simulink model "FB_Controller"  (R2018b)
settings: Solver=FixedStepDiscrete  StartTime=0.0  StopTime=50  FixedStep=1  MaxStep=1  RelTol=1e-3
values from neighbouring files (symbols this model uses):
  read_input_code = uint8(2)    [setup.m]
  timeout = int32(50)    [setup.m]
  write_output_code = uint8(4)    [setup.m]
undefined symbols (not defined in the file or in its folder): sldvsubsys
libraries: sldvlib x11, simulink x4, hdlsllib x3, simulink_extras x1
settings Model: PauseTimes=16.5  Creator=gauthamsm  LastModifiedBy=gauthamsm
settings DebuggingCC: IntegerOverflowMsg=error  IntegerSaturationMsg=error
settings ConfigComp: DVMode=PropertyProving  DVTestSuiteOptimization=CombinedObjectives (Nonlinear Extended)  DVDetectOutOfBounds=on

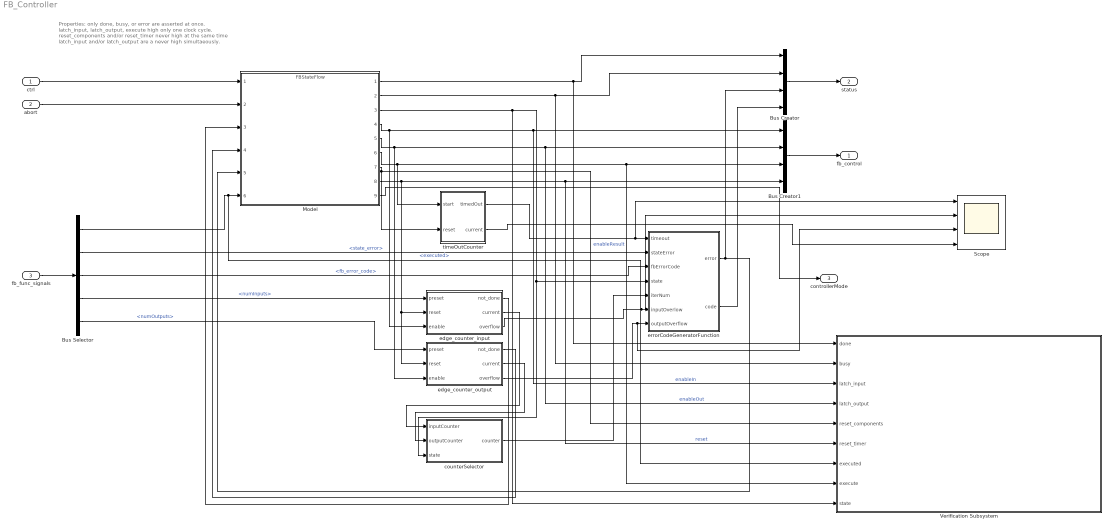
== system FB_Controller ==
  note: Properties:
      | only done, busy, or error are asserted at once.
      | latch_input, latch_output, execute high only one clock cycle.
      | reset_components and/or reset_timer never high at the same time latch_input and/or latch_output are a never high simultaeously.
  ctrl : Inport  RequirementInfo={} %GIDa_eee56b84_8a81_4d0c_8bf5_519b6d3ee13a  OutDataTypeStr=boolean
  abort : Inport  RequirementInfo={} %GIDa_f7a011da_777c_48fa_ab6a_d93ba2b9ac0e  Port=2  OutDataTypeStr=boolean
  fb_func_signals : Inport  RequirementInfo={} %GIDa_558a3938_4bec_4c5e_9357_eecde6866582  Port=3  OutDataTypeStr=Bus: fb_functions_out
  Bus Creator : BusCreator  RequirementInfo={} %GIDa_5b43234e_00ef_49d3_92d1_0649bce15cf8  Inputs=4  OutDataTypeStr=Bus: fb_status
  Bus Creator1 : BusCreator  RequirementInfo={} %GIDa_2879ab44_2c47_481b_b9a6_000ecd94b36b  Inputs=4  OutDataTypeStr=Bus: fb_control
  Bus Selector : BusSelector  RequirementInfo={} %GIDa_3f3a83a6_ae23_41f2_94a0_96f7ad6d1f78  OutputSignals=executed,state_error,fb_error_code,numInputs,numOutputs
  Model : ModelReference  RequirementInfo={} %GIDa_1daab9a8_dd2d_4e6d_9772_3109c5418e4f  ModelNameDialog=FBStateFlow.slx  SimulationMode=Normal  ModelReferenceVersion=1.25
  Scope : Scope  NumInputPorts=4
  Verification Subsystem : Subsystem  Tag=VerificationSubsystem  DisableCoverage=on  LoadFcn=sldvsubsys('check')  TreatAsAtomicUnit=on  SimViewingDevice=on  mask(VerificationSubsystem){}
      mask init:
      | sldvsubsys('maskInit');
      settings: CopyFcn=sldvsubsys('copy');  OpenFcn=open_system(gcb,'force');
      settings: PreSaveFcn=|
      | set_param(gcb,'SimViewingDevice','on');
      | sldvsubsys('check');
      mask Help: helpview(fullfile(docroot,'toolbox','sldv','sldv.map'),'verificationsubsystem')
      mask Display: image(imread('sldvicon_versubsys.png','BackGroundColor',[1 1 1]),'center');
  counterSelector : Subsystem  RequirementInfo={} %GIDa_611b34ef_a88f_49be_a0b4_a9f7defa758a  AncestorBlock=library/edge_counter
  edge_counter_input : Subsystem  AncestorBlock=library/edge_counter
  edge_counter_output : Subsystem  RequirementInfo={} %GIDa_3d032f53_0e8b_43fd_9dc3_9847963cb929  AncestorBlock=library/edge_counter
  errorCodeGeneratorFunction : Subsystem  RequirementInfo={} %GIDa_45c906d4_d4b7_4067_a1e4_bf9fe831da13
  timeOutCounter : Subsystem  RequirementInfo={} %GIDa_aee1d614_fa3b_47ff_99b8_964efb2c9353
  fb_control : Outport  RequirementInfo={} %GIDa_0f529c79_dd38_433f_9a7f_8a26aae76f29  OutDataTypeStr=Bus: fb_control
  status : Outport  RequirementInfo={} %GIDa_b0e0ce10_de37_4d28_9b9f_f8051855f138  Port=2  OutDataTypeStr=Bus: fb_status
  "controllerMode " : Outport  RequirementInfo={} %GIDa_91e3ca03_496d_47a8_8826_73fdaff52325  Port=3
  wires:
  edge_counter_input/3(overflow) -> Scope/2, errorCodeGeneratorFunction/6(inputOverlow)
  counterSelector/1(counter) -> errorCodeGeneratorFunction/5(iterNum)
  Bus Selector/2 -> errorCodeGeneratorFunction/2(stateError)  "<state_error>"
  Bus Selector/3 -> errorCodeGeneratorFunction/3(fbErrorCode)  "<fb_error_code>"
  Model/9 -> "controllerMode "/1
  Model/7 -> Verification Subsystem/5(reset_components), Verification Subsystem/6(reset_timer), Bus Creator1/4, edge_counter_output/2(reset), edge_counter_input/2(reset)  "reset"
  Bus Selector/5 -> edge_counter_output/1(preset)  "<numOutputs>"
  errorCodeGeneratorFunction/1(error) -> Model/5, Bus Creator/3
  Model/6 -> timeOutCounter/1(start), Verification Subsystem/8(execute), Bus Creator1/3  "enableResult"
  Bus Creator1/1 -> fb_control/1
  Model/2 -> Verification Subsystem/2(busy), Bus Creator/2
  Bus Creator/1 -> status/1
  Bus Selector/1 -> Verification Subsystem/7(executed), Model/6  "<executed>"
  Model/3 -> Verification Subsystem/9(state), errorCodeGeneratorFunction/4(state), counterSelector/3(state)
  edge_counter_output/2(current) -> counterSelector/2(outputCounter)
  edge_counter_input/2(current) -> counterSelector/1(inputCounter)
  Model/5 -> edge_counter_output/3(enable), Verification Subsystem/4(latch_output), Bus Creator1/2  "enableOut"
  timeOutCounter/1(timedOut) -> Scope/1, errorCodeGeneratorFunction/1(timeout)
  Bus Selector/4 -> edge_counter_input/1(preset)  "<numInputs>"
  edge_counter_output/1(not_done) -> Model/4
  Model/8 -> timeOutCounter/2(reset)
  fb_func_signals/1 -> Bus Selector/1
  abort/1 -> Model/2
  Model/1 -> Verification Subsystem/1(done), Bus Creator/1
  edge_counter_input/1(not_done) -> Model/3
  errorCodeGeneratorFunction/2(code) -> Bus Creator/4
  ctrl/1 -> Model/1
  Model/4 -> Verification Subsystem/3(latch_input), Bus Creator1/1, edge_counter_input/3(enable)  "enableIn"
  edge_counter_output/3(overflow) -> Scope/3, errorCodeGeneratorFunction/7(outputOverflow)
  timeOutCounter/2(current) -> Scope/4

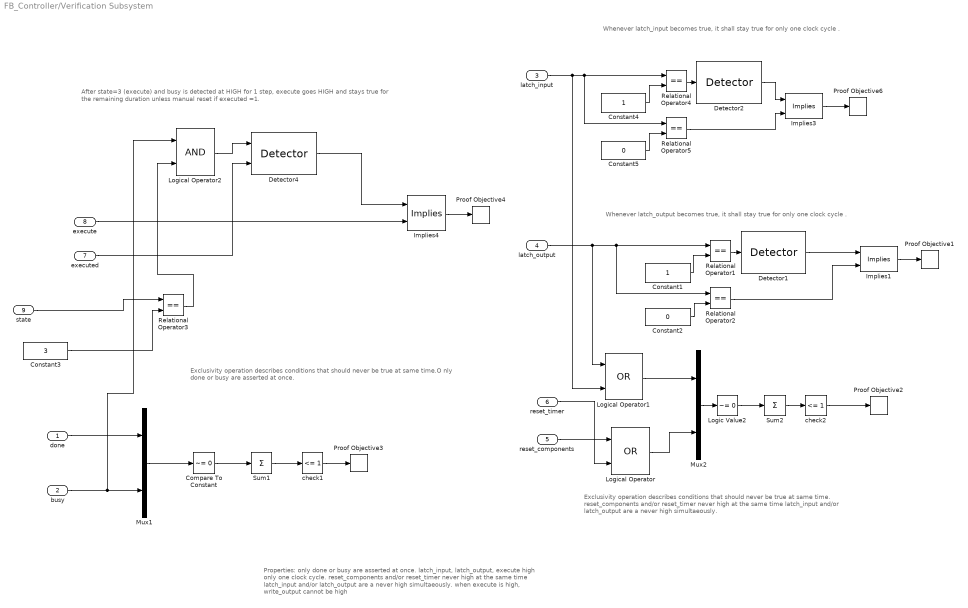
== system FB_Controller/Verification Subsystem ==
  note: Exclusivity operation describes conditions that should
      | never be true at same time.O nly done or busy are asserted at once.
  note: Properties:
      | only done or busy are asserted at once.
      | latch_input, latch_output, execute high only one clock cycle.
      | reset_components and/or reset_timer never high at the same time latch_input and/or latch_output are a never high simultaeously.
      | when execute is high, write_output cannot be high
  note: Whenever latch_output becomes true, it shall stay true for only one clock cycle .
  note: Whenever latch_input becomes true, it shall stay true for only one clock cycle .
  note: Exclusivity operation describes conditions that should
      | never be true at same time.
      | reset_components and/or reset_timer never high at the
      | same time latch_input and/or latch_output are a never high simultaeously.
  note: After state=3 (execute) and busy is detected at HIGH for 1  step, execute goes HIGH and stays true for
      | the remaining duration unless manual reset if executed =1.
  done : Inport
  busy : Inport  Port=2
  latch_input : Inport  Port=3
  latch_output : Inport  Port=4
  reset_components : Inport  Port=5
  reset_timer : Inport  Port=6
  executed : Inport  Port=7
  execute : Inport  Port=8
  state : Inport  Port=9
  Compare To Constant : simulink/Logic and Bit Operations/Compare To Constant  relop=~=  const=0  OutDataTypeStr=boolean
  Constant1 : Constant
  Constant2 : Constant  Value=0
  Constant3 : Constant  Value=3
  Constant4 : Constant
  Constant5 : Constant  Value=0
  Detector1 : sldvlib/Temporal Operators/Detector  reset=off  typ=Delayed Fixed Duration  in_hold=1  delay=0  out_hold=1
      settings: SourceProductName=Simulink Design Verifier  SourceProductBaseCode=DV
  Detector2 : sldvlib/Temporal Operators/Detector  reset=off  typ=Delayed Fixed Duration  in_hold=1  delay=0  out_hold=1
      settings: SourceProductName=Simulink Design Verifier  SourceProductBaseCode=DV
  Detector4 : sldvlib/Temporal Operators/Detector  reset=on  typ=Delayed Fixed Duration  in_hold=1  delay=0  out_hold=1
      settings: SourceProductName=Simulink Design Verifier  SourceProductBaseCode=DV
  Implies1 : sldvlib/Verification Utilities/Implies
      settings: SourceProductName=Simulink Design Verifier  SourceProductBaseCode=DV
  Implies3 : sldvlib/Verification Utilities/Implies
      settings: SourceProductName=Simulink Design Verifier  SourceProductBaseCode=DV
  Implies4 : sldvlib/Verification Utilities/Implies
      settings: SourceProductName=Simulink Design Verifier  SourceProductBaseCode=DV
  Logic Value2 : simulink/Logic and Bit Operations/Compare To Zero  relop=~=  OutDataTypeStr=uint8  ZeroCross=off
  Logical Operator : Logic  Operator=OR  AllPortsSameDT=off  OutDataTypeStr=boolean
  Logical Operator1 : Logic  Operator=OR  AllPortsSameDT=off  OutDataTypeStr=boolean
  Logical Operator2 : Logic  AllPortsSameDT=off  OutDataTypeStr=boolean
  Mux1 : Mux  Inputs=2
  Mux2 : Mux  Inputs=2
  Proof Objective{1..4,6} (5 alike) : sldvlib/Objectives and Constraints/Proof Objective  enabled=on  customAVTBlockType=Proof Objective  intervals=true  dispValues=on  outEnabled=off  enableStopSim=off
      settings: AttributesFormatString=%<intervals>  SourceProductName=Simulink Design Verifier  SourceProductBaseCode=DV
  Relational Operator{1..5} (5 alike) : RelationalOperator  Operator===  OutDataTypeStr=boolean  RndMeth=Nearest
  Sum1 : Sum  Inputs=+  AccumDataTypeStr=uint8  OutDataTypeStr=uint8  SaturateOnIntegerOverflow=on
  Sum2 : Sum  Inputs=+  AccumDataTypeStr=uint8  OutDataTypeStr=uint8  SaturateOnIntegerOverflow=on
  check1 : simulink/Logic and Bit Operations/Compare To Constant  relop=<=  const=1  OutDataTypeStr=boolean  ZeroCross=off
  check2 : simulink/Logic and Bit Operations/Compare To Constant  relop=<=  const=1  OutDataTypeStr=boolean  ZeroCross=off
  wires:
  Compare To Constant/1 -> Sum1/1
  Sum1/1 -> check1/1
  done/1 -> Mux1/1
  Logic Value2/1 -> Sum2/1
  check2/1 -> Proof Objective2/1
  Sum2/1 -> check2/1
  Mux2/1 -> Logic Value2/1
  reset_components/1 -> Logical Operator/1
  reset_timer/1 -> Logical Operator/2
  Logical Operator1/1 -> Mux2/1
  Logical Operator/1 -> Mux2/2
  Relational Operator5/1 -> Implies3/2
  Constant4/1 -> Relational Operator4/2
  Constant5/1 -> Relational Operator5/2
  Implies3/1 -> Proof Objective6/1
  latch_input/1 -> Logical Operator1/2, Relational Operator5/1, Relational Operator4/1
  Detector2/1 -> Implies3/1
  Relational Operator4/1 -> Detector2/1
  latch_output/1 -> Relational Operator2/1, Relational Operator1/1, Logical Operator1/1
  Relational Operator1/1 -> Detector1/1
  Detector1/1 -> Implies1/1
  Constant1/1 -> Relational Operator1/2
  Constant2/1 -> Relational Operator2/2
  Implies1/1 -> Proof Objective1/1
  Relational Operator2/1 -> Implies1/2
  Logical Operator2/1 -> Detector4/1
  state/1 -> Relational Operator3/1
  Constant3/1 -> Relational Operator3/2
  Detector4/1 -> Implies4/1
  Implies4/1 -> Proof Objective4/1
  executed/1 -> Detector4/2
  Relational Operator3/1 -> Logical Operator2/2
  execute/1 -> Implies4/2
  busy/1 -> Logical Operator2/1, Mux1/2
  Mux1/1 -> Compare To Constant/1
  check1/1 -> Proof Objective3/1

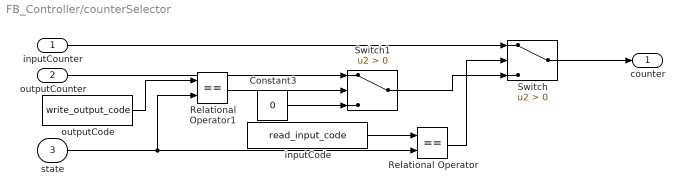
== system FB_Controller/counterSelector ==
  inputCounter : Inport  RequirementInfo={} %GIDa_32673686_52f4_4205_a851_289b051ccb74
  outputCounter : Inport  RequirementInfo={} %GIDa_2bec27ec_9a5e_4d6f_a356_5cfaf745abff  Port=2
  state : Inport  RequirementInfo={} %GIDa_e53867f6_75b4_4b77_a450_934a48bb110d  Port=3
  Constant3 : Constant  RequirementInfo={} %GIDa_1fd085bb_7886_48ea_b698_9ea29fa2839f  Value=0  SampleTime=-1
  Relational Operator : RelationalOperator  RequirementInfo={} %GIDa_bab68883_1a8c_4354_9c05_0d4b7d901c58  Operator===  OutDataTypeStr=boolean  RndMeth=Nearest
  Relational Operator1 : RelationalOperator  RequirementInfo={} %GIDa_dc0544f8_80ca_4437_b208_c176972d6f15  Operator===  OutDataTypeStr=boolean  RndMeth=Nearest
  Switch : Switch  RequirementInfo={} %GIDa_45fb47f3_43db_4c17_bb19_9a61542264b4  Criteria=u2 > Threshold
  Switch1 : Switch  RequirementInfo={} %GIDa_5ba4db5e_340a_4c29_8263_ec20f82287c5  Criteria=u2 > Threshold
  inputCode : Constant  RequirementInfo={} %GIDa_b12fcaa5_8f72_40cc_987a_eb3173891b33  Value=read_input_code  SampleTime=-1
  outputCode : Constant  RequirementInfo={} %GIDa_a763eaef_93a5_40bd_91a8_2354a77a0e84  Value=write_output_code  SampleTime=-1
  counter : Outport  RequirementInfo={} %GIDa_4e060737_4dca_4352_9628_00158348805d
  wires:
  Switch1/1 -> Switch/3
  Constant3/1 -> Switch1/3
  Relational Operator/1 -> Switch/2
  Relational Operator1/1 -> Switch1/2
  outputCode/1 -> Relational Operator1/1
  Switch/1 -> counter/1
  inputCode/1 -> Relational Operator/1
  outputCounter/1 -> Switch1/1
  inputCounter/1 -> Switch/1
  state/1 -> Relational Operator/2, Relational Operator1/2

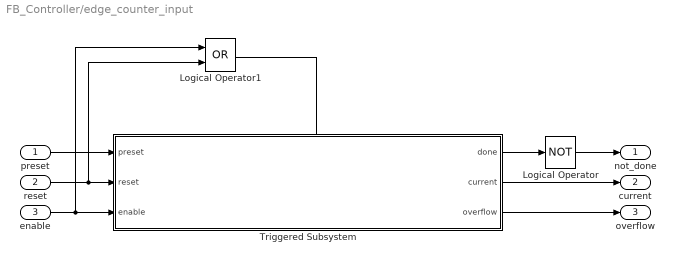
== system FB_Controller/edge_counter_input ==
  preset : Inport
  reset : Inport  Port=2
  enable : Inport  Port=3
  Logical Operator : Logic  Operator=NOT  AllPortsSameDT=off  OutDataTypeStr=boolean
  Logical Operator1 : Logic  Operator=OR  AllPortsSameDT=off  OutDataTypeStr=boolean
  Triggered Subsystem : Subsystem  TreatAsAtomicUnit=on
  not_done : Outport
  current : Outport  Port=2
  overflow : Outport  Port=3
  wires:
  Logical Operator/1 -> not_done/1
  Triggered Subsystem/3(overflow) -> overflow/1
  Triggered Subsystem/2(current) -> current/1
  Triggered Subsystem/1(done) -> Logical Operator/1
  reset/1 -> Logical Operator1/2, Triggered Subsystem/2(reset)
  preset/1 -> Triggered Subsystem/1(preset)
  enable/1 -> Logical Operator1/1, Triggered Subsystem/3(enable)
  Logical Operator1/1 -> ?

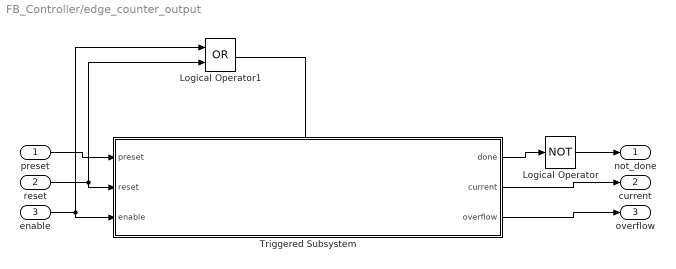
== system FB_Controller/edge_counter_output ==
  preset : Inport  RequirementInfo={} %GIDa_227c2d3f_4628_4bbd_8c59_6ffaaa625778
  reset : Inport  RequirementInfo={} %GIDa_27945d62_463f_47c7_99b2_44b5db58e10e  Port=2
  enable : Inport  RequirementInfo={} %GIDa_189158c6_a714_4286_94d9_6e9d413cd09a  Port=3
  Logical Operator : Logic  RequirementInfo={} %GIDa_403dfc36_36fa_4f2a_bf18_a3551986af17  Operator=NOT  AllPortsSameDT=off  OutDataTypeStr=boolean
  Logical Operator1 : Logic  RequirementInfo={} %GIDa_c349ede8_73ab_4b55_9980_852154509574  Operator=OR  AllPortsSameDT=off  OutDataTypeStr=boolean
  Triggered Subsystem : Subsystem  RequirementInfo={} %GIDa_890350e1_922d_43a9_8892_ccd60a6bc9d9  TreatAsAtomicUnit=on
  not_done : Outport  RequirementInfo={} %GIDa_9c82c7be_3521_4def_b4bd_66e97367d995
  current : Outport  RequirementInfo={} %GIDa_0a7e95c2_2feb_4c6f_994f_f883f6a324cd  Port=2
  overflow : Outport  RequirementInfo={} %GIDa_00300313_88ae_4fb1_99fc_d31435c6cebc  Port=3
  wires:
  Logical Operator1/1 -> ?
  Logical Operator/1 -> not_done/1
  Triggered Subsystem/3(overflow) -> overflow/1
  Triggered Subsystem/2(current) -> current/1
  Triggered Subsystem/1(done) -> Logical Operator/1
  reset/1 -> Logical Operator1/2, Triggered Subsystem/2(reset)
  preset/1 -> Triggered Subsystem/1(preset)
  enable/1 -> Logical Operator1/1, Triggered Subsystem/3(enable)

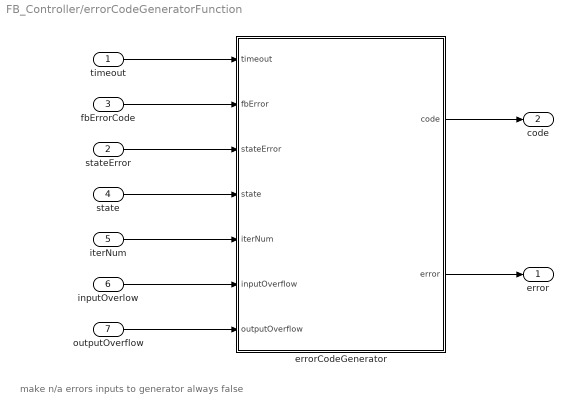
== system FB_Controller/errorCodeGeneratorFunction ==
  note: make n/a errors inputs to generator always false
  timeout : Inport  RequirementInfo={} %GIDa_592c4668_4c68_463a_9a61_204f4080ed5b
  stateError : Inport  RequirementInfo={} %GIDa_be401f4e_e636_4141_8e01_12413cb729fe  Port=2
  fbErrorCode : Inport  RequirementInfo={} %GIDa_678ca061_bccd_4db4_85e6_74696e7d13cc  Port=3
  state : Inport  RequirementInfo={} %GIDa_7334bf15_6798_46b4_b3a0_9a68d9a9b9af  Port=4
  iterNum : Inport  RequirementInfo={} %GIDa_18843df4_3017_43a6_b24d_98337e2131b3  Port=5
  inputOverlow : Inport  RequirementInfo={} %GIDa_db239c11_6a88_4867_aaa5_adc81db3fd5b  Port=6
  outputOverflow : Inport  RequirementInfo={} %GIDa_fd601b08_468e_47b9_a25b_f3ee506c1818  Port=7
  errorCodeGenerator : MATLAB Function  RequirementInfo={} %GIDa_9c826adc_eb18_4b06_879e_82b7a72f9eb9  TreatAsAtomicUnit=on
  error : Outport  RequirementInfo={} %GIDa_e2919ecb_fa8d_4c70_b433_57dfed1dfb70  OutDataTypeStr=boolean
  code : Outport  RequirementInfo={} %GIDa_4435a261_0dcc_4353_8c2c_75730bbec3dd  Port=2  OutDataTypeStr=uint32
  wires:
  errorCodeGenerator/1(code) -> code/1
  timeout/1 -> errorCodeGenerator/1(timeout)
  stateError/1 -> errorCodeGenerator/3(stateError)
  errorCodeGenerator/2(error) -> error/1
  fbErrorCode/1 -> errorCodeGenerator/2(fbError)
  state/1 -> errorCodeGenerator/4(state)
  iterNum/1 -> errorCodeGenerator/5(iterNum)
  outputOverflow/1 -> errorCodeGenerator/7(outputOverflow)
  inputOverlow/1 -> errorCodeGenerator/6(inputOverflow)

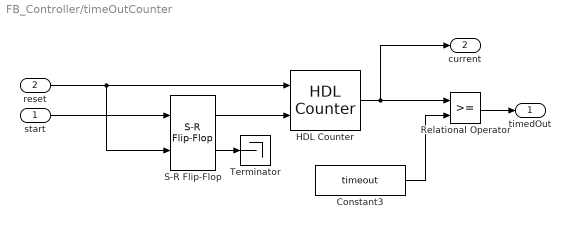
== system FB_Controller/timeOutCounter ==
  start : Inport  RequirementInfo={} %GIDa_df429725_c845_43eb_82b6_1a9fc51af239
  reset : Inport  RequirementInfo={} %GIDa_8b52eaba_e55b_4d20_afcb_755572acbc00  Port=2
  Constant3 : Constant  RequirementInfo={} %GIDa_97a67ee4_c9a2_479a_8d0a_01ac69458071  Value=timeout
  HDL Counter : hdlsllib/Sources/HDL Counter  RequirementInfo={} %GIDa_5945bfbb_e971_4862_8878_8c774b6a0469  CountType=Count limited  CountInit=0  CountStep=1  CountMax=255  CountFromType=Initial value  CountFrom=0  CountResetPort=on  CountLoadPort=off  CountEnbPort=on  CountDirPort=off  CountDataType=Unsigned  CountWordLen=8  CountFracLen=0  CountSampTime=1
      settings: SourceProductBaseCode=HD
  Relational Operator : RelationalOperator  RequirementInfo={} %GIDa_56f07c8d_32e5_47d3_9fbc_d993d5dbe5ed  OutDataTypeStr=boolean  RndMeth=Simplest
  S-R Flip-Flop : simulink_extras/Flip Flops/S-R Flip-Flop  RequirementInfo={} %GIDa_1aeaf069_acb8_4409_976c_462a8a3b563f  initial_condition=0
  Terminator : Terminator
      settings: RequirementInfo={} %GIDa_fdfab7f2_cb11_458a_83af_c73f2b469561
  timedOut : Outport  RequirementInfo={} %GIDa_6bf235d4_69dd_42f8_8435_57ce111961ff
  current : Outport  Port=2
  wires:
  S-R Flip-Flop/1 -> HDL Counter/2
  Relational Operator/1 -> timedOut/1
  HDL Counter/1 -> current/1, Relational Operator/1
  S-R Flip-Flop/2 -> Terminator/1
  Constant3/1 -> Relational Operator/2
  reset/1 -> HDL Counter/1, S-R Flip-Flop/2
  start/1 -> S-R Flip-Flop/1

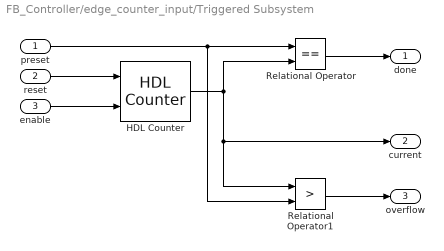
== system FB_Controller/edge_counter_input/Triggered Subsystem ==
  preset : Inport
  reset : Inport  Port=2
  enable : Inport  Port=3
  HDL Counter : hdlsllib/Sources/HDL Counter  CountType=Free running  CountInit=0  CountStep=1  CountMax=25  CountFromType=Initial value  CountFrom=0  CountResetPort=on  CountLoadPort=off  CountEnbPort=on  CountDirPort=off  CountDataType=Unsigned  CountWordLen=8  CountFracLen=0  CountSampTime=1
      settings: SourceProductBaseCode=HD
  Relational Operator : RelationalOperator  Operator===  OutDataTypeStr=boolean  RndMeth=Simplest
  Relational Operator1 : RelationalOperator  Operator=>  OutDataTypeStr=boolean  RndMeth=Simplest
  done : Outport
  current : Outport  Port=2
  overflow : Outport  Port=3
  wires:
  enable/1 -> HDL Counter/2
  reset/1 -> HDL Counter/1
  Relational Operator/1 -> done/1
  preset/1 -> Relational Operator/1, Relational Operator1/2
  HDL Counter/1 -> Relational Operator1/1, current/1, Relational Operator/2
  Relational Operator1/1 -> overflow/1

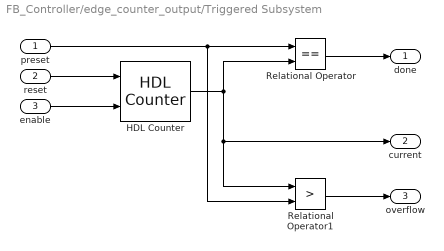
== system FB_Controller/edge_counter_output/Triggered Subsystem ==
  preset : Inport  RequirementInfo={} %GIDa_b710cb4c_1a9b_4aa6_a340_ff9a9f35ab90
  reset : Inport  RequirementInfo={} %GIDa_245e9dd0_769b_4afd_9378_60a64219b7da  Port=2
  enable : Inport  RequirementInfo={} %GIDa_a0796e81_05b5_4975_ab28_5f372ca60b9a  Port=3
  HDL Counter : hdlsllib/Sources/HDL Counter  RequirementInfo={} %GIDa_521b203c_1ddc_4b5e_b202_b0f4a6ced66d  CountType=Free running  CountInit=0  CountStep=1  CountMax=25  CountFromType=Initial value  CountFrom=0  CountResetPort=on  CountLoadPort=off  CountEnbPort=on  CountDirPort=off  CountDataType=Unsigned  CountWordLen=8  CountFracLen=0  CountSampTime=1
      settings: SourceProductBaseCode=HD
  Relational Operator : RelationalOperator  RequirementInfo={} %GIDa_d52915d4_5375_4923_ad44_649f0ba11564  Operator===  OutDataTypeStr=boolean  RndMeth=Simplest
  Relational Operator1 : RelationalOperator  RequirementInfo={} %GIDa_311999bd_494b_42c7_ab1c_936d49aa51a0  Operator=>  OutDataTypeStr=boolean  RndMeth=Simplest
  done : Outport  RequirementInfo={} %GIDa_74cc0173_bb8a_45cd_a590_689ac822598d
  current : Outport  RequirementInfo={} %GIDa_81cb726a_9280_49f0_8878_7d7330bfee39  Port=2
  overflow : Outport  RequirementInfo={} %GIDa_1286965d_7bb3_4401_973e_8de0bca22ec2  Port=3
  wires:
  enable/1 -> HDL Counter/2
  reset/1 -> HDL Counter/1
  Relational Operator/1 -> done/1
  preset/1 -> Relational Operator/1, Relational Operator1/2
  HDL Counter/1 -> Relational Operator1/1, current/1, Relational Operator/2
  Relational Operator1/1 -> overflow/1

== matlab function FB_Controller/errorCodeGeneratorFunction/errorCodeGenerator ==
  data: timeout input; fbError input; code output; stateError input; state input; iterNum input; inputOverflow input; outputOverflow input; error output; mask parameter
function [code,error] = fcn(timeout, fbError, stateError, state, iterNum, inputOverflow, outputOverflow, mask)

%#codegen
% FB Error Code Design (6/21/2018)
%       State  Iter#   Error#(&flags)
% Page | 0-15 | 0-15 |             |
% Bits |  4   |  6   |      22     |

% Defines the codes
errorCode = uint32(0);
stateCode = uint32(0);
iterCode = uint32(0);
code = uint32(0);

% Set the error bits (multiply with mask for bools, AND with mask for ints)
% Binary Inputs
errorCode = bitor(errorCode,mask.error.timeoutBit*uint32(timeout));
errorCode = bitor(errorCode,mask.error.stateErrorBit*uint32(stateError));
errorCode = bitor(errorCode,mask.error.inputOverflowBit*uint32(inputOverflow));
errorCode = bitor(errorCode,mask.error.outputOverflowBit*uint32(outputOverflow));
% Integer inputs
errorCode = bitor(errorCode,bitand(mask.error.divideByZeroBit,uint32(fbError)));
errorCode = bitor(errorCode,bitand(mask.error.overflowBit,uint32(fbError)));
errorCode = bitor(errorCode,bitand(mask.error.underflowBit,uint32(fbError)));
errorCode = bitsll(errorCode,mask.errorBitsShift); % Shifts the state code to the proper location
errorCode = bitand(errorCode,mask.errorBits); % ANDs it with the error mask for safety

% Set the state bits
stateCode = bitsll(uint32(state),mask.stateBitsShift); % Shifts the state code to the proper location
stateCode = bitand(stateCode,mask.stateBits); % ANDs it with the state mask for safety

% Set the iteration count bits
iterCode = bitsll(uint32(iterNum),mask.iterNumBitsShift); % Shifts the iteration code to the proper location
iterCode = bitand(iterCode,mask.iterNumBits); % ANDs it with the iteration mask for safety

code = bitor(code,errorCode);
code = bitor(code,stateCode);
code = bitor(code,iterCode);

% Give binary output for State machine input
if errorCode==uint32(0)
    error = false;
else
    error = true;
end

end
